simulink model "Tarea5R"  (R2020b)
settings: Solver=VariableStepAuto  StartTime=0.0  StopTime=10.0  RelTol=1e-3
settings Model: Creator=cesar  LastModifiedBy=cesar

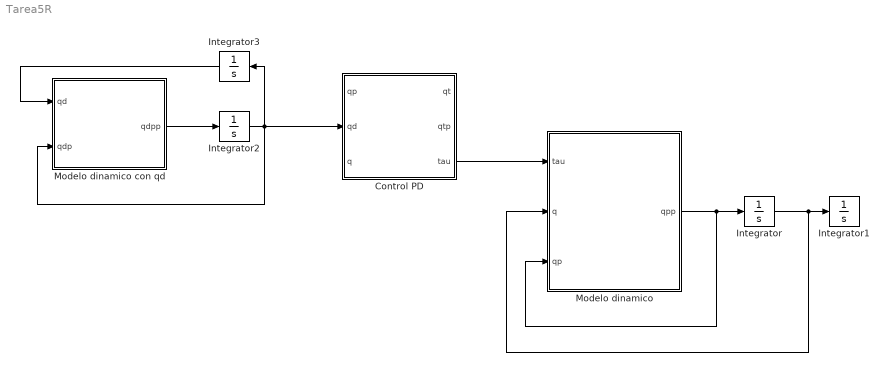
== system Tarea5R ==
  Control PD : MATLAB Function  TreatAsAtomicUnit=on
  Integrator{,1..3} (4 alike) : Integrator
  Modelo dinamico : MATLAB Function  TreatAsAtomicUnit=on
  Modelo dinamico con qd : MATLAB Function  TreatAsAtomicUnit=on
  wires:
  Modelo dinamico/1(qpp) -> Modelo dinamico/3(qp), Integrator/1
  Integrator/1 -> Modelo dinamico/2(q), Integrator1/1
  Control PD/3(tau) -> Modelo dinamico/1(tau)
  Modelo dinamico con qd/1(qdpp) -> Integrator2/1
  Integrator2/1 -> Integrator3/1, Modelo dinamico con qd/2(qdp), Control PD/2(qd)
  Integrator3/1 -> Modelo dinamico con qd/1(qd)

== matlab function Tarea5R/Control PD ==
  data: qt output; qtp output; qp input; tau output; qd input; q input
function [qt, qtp, tau]  = fcn(qp,qd,q)
kp=0.25;
mgl=1;
qd=pi/2;
kv=0.5;

qt= qd -q;
g = mgl*sin(q);

tau = kp*qt + kv*qp + g;

== matlab function Tarea5R/Modelo dinamico ==
  data: tau input; qpp output; q input; qp input

function qpp = fcn(tau, q, qp)

ml2 = 1;
mgl = 1;

qpp = (tau-mgl*sin(q))/ml2;

== matlab function Tarea5R/Modelo dinamico con qd ==
  data: qdpp output; qd input; qdp input
function qdpp = fcn(qd, qdp)

J=5;
ml2=1;

Jl=J+ml2;
M=Jl;

qdpp = 0;
